simulink model "Spracherkennungslx"  (R2020a)
settings: Solver=VariableStepAuto  StartTime=0.0  StopTime=inf  RelTol=1e-3
libraries: audiomeasurements x1
settings Model: Creator=alf  LastModifiedBy=alf
settings SFSimCC: SimUserSources=test.cpp  CustomCodeUndefinedFunction=ThrowError

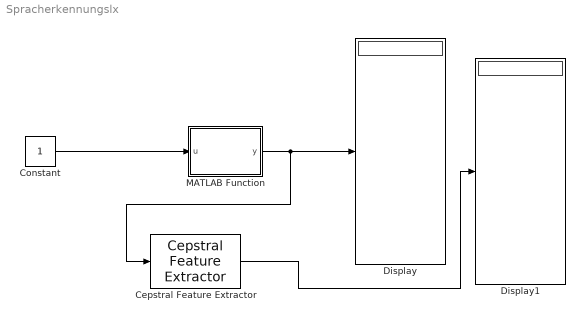
== system Spracherkennungslx ==
  Cepstral Feature Extractor : audiomeasurements/Cepstral Feature Extractor  FilterBank=Mel  InputDomain=Time  NumCoeffs=13  Rectification=Log  InheritFFTLength=on  FFTLength=[]  LogEnergy=Append  OutputDelta=off  OutputDeltaDelta=off  InheritSampleRate=off  SampleRate=16000  SimulateUsing=Code generation  FrequencyRange=[ 50, 8000 ]  BandEdges=[133.33333333333334 200 266.66666666666669 333.33333333333337 400 466.66666666666674 533.33333333333337 600 666.66666666666674 733.33333333333337 800.00000000000011 866.66666666666674 933.33333333333337 999.75894666666659 1070.9120908286172 1147.1292256065171 1228.7707567317004 1316.2227401195225 1409.8987074006509 1510.2416213759673 1617.725970641781 1732.8600132901477 1856.1881802940113 1988.29364994199 2129.8011054964563 2281.3796891149705 2443.7461660031895 2617.6683137614859 2803.9685529523849 3003.5278360565717 3217.2898132070686 3446.2652943999592 3691.5370292819921 3954.2648271171001 4235.6910411424715 4537.1464432478933 4860.0565167577788 5205.9481970723846 5576.4570920424849 5973.3352162202755 6398.4592755592366 6853.83954173857]  FilterBankDesignDomain=Hz  FilterBankNormalization=Bandwidth
      settings: SourceProductBaseCode=AU
  Constant : Constant
  Display : Display
  Display1 : Display
  MATLAB Function : MATLAB Function  TreatAsAtomicUnit=on
  wires:
  Constant/1 -> MATLAB Function/1(u)
  MATLAB Function/1(y) -> Cepstral Feature Extractor/1, Display/1
  Cepstral Feature Extractor/1 -> Display1/1

== matlab function Spracherkennungslx/MATLAB Function ==
  data: u input; y output
function y = fcn(u)
    u1 = cast(zeros(1,10),'single');
    b = 0;
    y = cast(zeros(1,10),'single');
    coder.extrinsic('test_mex');
    u1 = test_mex(b);
y = u1;
